simulink model "JABS"  (R2018b)
settings: Solver=FixedStepDiscrete  StartTime=0.0  StopTime=10.0  FixedStep=0.01  RelTol=1e-3
(part 2 of 2)

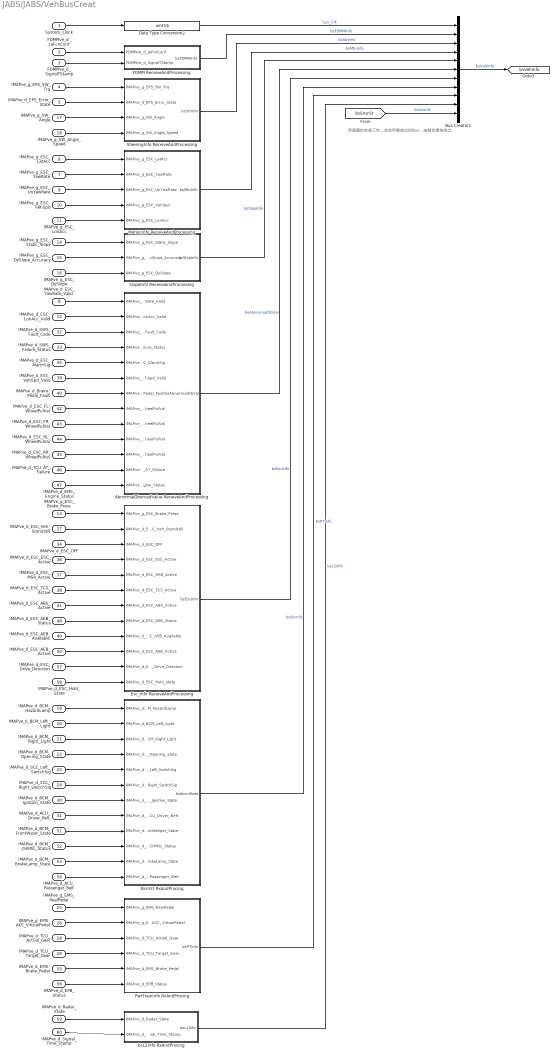
== system JABS/JABS/VehBusCreat ==
  note: 传感器的本身工作状态所集成出的Bus，由融合模块给出
  System_Clock : Inport
  FDMMve_d_JaFcnConf : Inport  Port=2
  FDMMve_d_SignalTStamp : Inport  Port=3
  IMAPve_g_EPS_SW_Trq : Inport  Port=4
  IMAPve_d_EPS_Error_State : Inport  Port=5
  IMAPve_g_ESC_LatAcc : Inport  Port=6
  IMAPve_g_ESC_YawRate : Inport  Port=7
  IMAPve_d_ESC_YawRate_Valid : Inport  Port=8
  IMAPve_g_ESC_UnYawRate : Inport  Port=9
  IMAPve_g_ESC_VehSpd : Inport  Port=10
  IMAPve_g_ESC_LonAcc : Inport  Port=11
  IMAPve_d_ESC_LonAcc_Valid : Inport  Port=12
  IMAPve_g_ESC_Brake_Press : Inport  Port=13
  IMAPve_g_ESC_Static_Slope : Inport  Port=14
  IMAPve_g_ESC_DySlope_Accuracy : Inport  Port=15
  IMAPve_g_ESC_DySlope : Inport  Port=16
  IMAPve_g_SW_Angle : Inport  Port=17
  IMAPve_g_SW_Angle_Speed : Inport  Port=18
  IMAPve_d_BCM_HazardLamp : Inport  Port=19
  IMAPve_d_BCM_Left_Light : Inport  Port=20
  IMAPve_d_BCM_Right_Light : Inport  Port=21
  IMAPve_d_BCM_Opening_State : Inport  Port=22
  IMAPve_d_SCC_Left_SwitchSig : Inport  Port=23
  IMAPve_d_SCC_Right_SwitchSig : Inport  Port=24
  IMAPve_g_EMS_RealPedal : Inport  Port=25
  IMAPve_g_EMS_ACC_VirtualPedal : Inport  Port=26
  IMAPve_d_ESC_Veh_Standstill : Inport  Port=27
  IMAPve_d_TCU_Actual_Gear : Inport  Port=28
  IMAPve_d_TCU_Target_Gear : Inport  Port=29
  IMAPve_d_BCM_Ignition_State : Inport  Port=30
  IMAPve_d_ACU_Driver_Belt : Inport  Port=31
  IMAPve_d_SWS_Fault_Code : Inport  Port=32
  IMAPve_d_SWS_Failure_Status : Inport  Port=33
  IMAPve_d_ESC_OFF : Inport  Port=34
  IMAPve_d_ESC_AlarmSig : Inport  Port=35
  IMAPve_d_ESC_ESC_Active : Inport  Port=36
  IMAPve_d_ESC_MSR_Active : Inport  Port=37
  IMAPve_d_ESC_TCS_Active : Inport  Port=38
  IMAPve_d_ESC_VehSpd_Valid : Inport  Port=39
  IMAPve_d_Brake_Pedal_Fault : Inport  Port=40
  IMAPve_d_ESC_ABS_Active : Inport  Port=41
  IMAPve_d_ESC_FL_WheelPulVal : Inport  Port=42
  IMAPve_d_ESC_FR_WheelPulVal : Inport  Port=43
  IMAPve_d_ESC_RL_WheelPulVal : Inport  Port=44
  IMAPve_d_ESC_RR_WheelPulVal : Inport  Port=45
  IMAPve_d_TCU_AT_Failure : Inport  Port=46
  IMAPve_d_EMS_Engine_Status : Inport  Port=47
  IMAPve_d_ESC_AEB_Status : Inport  Port=48
  IMAPve_d_ESC_AEB_Available : Inport  Port=49
  IMAPve_d_ESC_AEB_Active : Inport  Port=50
  IMAPve_d_BCM_FrontWiper_State : Inport  Port=51
  IMAPve_d_BCM_CHMSL_Status : Inport  Port=52
  IMAPve_d_BCM_BrakeLamp_State : Inport  Port=53
  IMAPve_d_ACU_Passenger_Belt : Inport  Port=54
  IMAPve_d_EMS_Brake_Pedal : Inport  Port=55
  IMAPve_d_EPB_Status : Inport  Port=56
  IMAPve_d_ESC_Drive_Direction : Inport  Port=57
  IMAPve_d_ESC_Hold_State : Inport  Port=58
  IMAPve_d_Radar_State : Inport  Port=59
  IMAPve_d_Signal_Time_Stamp : Inport  Port=60
  AbnormalObervedValue ReceiveAndProcessing : Subsystem
  BcmSt RxAndProcing : Subsystem
  Bus Creator1 : BusCreator  Inputs=11
  Data Type Conversion2 : DataTypeConversion  OutDataTypeStr=uint16
  Esc_Info ReceiveAndProcessing : Subsystem
  FDMM ReceiveAndProcessing : Subsystem
  MotionInfo ReceiveAndProcessing : Subsystem
  PwrTrainInfo RxAndProcing : Subsystem
  SlopeInfo ReceiveAndProcessing : Subsystem
  SteeringInfo ReceiveAndProcessing : Subsystem
  bsL2Info RxAndProcing : Subsystem
  tag scope: bsVehInfo=global
  wires:
  System_Clock/1 -> Data Type Conversion2/1
  IMAPve_d_EMS_Engine_Status/1 -> AbnormalObervedValue ReceiveAndProcessing/13(IMAPve_d_EMS_Engine_Status)
  IMAPve_d_TCU_AT_Failure/1 -> AbnormalObervedValue ReceiveAndProcessing/12(IMAPve_d_TCU_AT_Failure)
  SteeringInfo ReceiveAndProcessing/1(bsStrInfo) -> Bus Creator1/3  "bsStrInfo"
  IMAPve_d_Brake_Pedal_Fault/1 -> AbnormalObervedValue ReceiveAndProcessing/7(IMAPve_d_Brake_Pedal_Fault)
  IMAPve_d_ESC_FL_WheelPulVal/1 -> AbnormalObervedValue ReceiveAndProcessing/8(IMAPve_d_ESC_FL_WheelPulVal)
  IMAPve_g_SW_Angle/1 -> SteeringInfo ReceiveAndProcessing/3(IMAPve_g_SW_Angle)
  Esc_Info ReceiveAndProcessing/1(bsEscInfo) -> Bus Creator1/7  "bsEscInfo"
  IMAPve_d_EPS_Error_State/1 -> SteeringInfo ReceiveAndProcessing/2(IMAPve_d_EPS_Error_State)
  IMAPve_d_ESC_VehSpd_Valid/1 -> AbnormalObervedValue ReceiveAndProcessing/6(IMAPve_d_ESC_VehSpd_Valid)
  IMAPve_d_ESC_RL_WheelPulVal/1 -> AbnormalObervedValue ReceiveAndProcessing/10(IMAPve_d_ESC_RL_WheelPulVal)
  IMAPve_d_ESC_AlarmSig/1 -> AbnormalObervedValue ReceiveAndProcessing/5(IMAPve_d_ESC_AlarmSig)
  IMAPve_d_ESC_FR_WheelPulVal/1 -> AbnormalObervedValue ReceiveAndProcessing/9(IMAPve_d_ESC_FR_WheelPulVal)
  IMAPve_d_SWS_Failure_Status/1 -> AbnormalObervedValue ReceiveAndProcessing/4(IMAPve_d_SWS_Failure_Status)
  PwrTrainInfo RxAndProcing/1(bsPTInfo) -> Bus Creator1/9  "bsPTInfo"
  MotionInfo ReceiveAndProcessing/1(bsMtnInfo) -> Bus Creator1/4  "bsMtnInfo"
  IMAPve_g_SW_Angle_Speed/1 -> SteeringInfo ReceiveAndProcessing/4(IMAPve_g_SW_Angle_Speed)
  IMAPve_d_ESC_RR_WheelPulVal/1 -> AbnormalObervedValue ReceiveAndProcessing/11(IMAPve_d_ESC_RR_WheelPulVal)
  IMAPve_g_EMS_RealPedal/1 -> PwrTrainInfo RxAndProcing/1(IMAPve_g_EMS_RealPedal)
  IMAPve_g_EMS_ACC_VirtualPedal/1 -> PwrTrainInfo RxAndProcing/2(IMAPve_g_EMS_ACC_VirtualPedal)
  IMAPve_d_TCU_Actual_Gear/1 -> PwrTrainInfo RxAndProcing/3(IMAPve_d_TCU_Actual_Gear)
  IMAPve_d_SWS_Fault_Code/1 -> AbnormalObervedValue ReceiveAndProcessing/3(IMAPve_d_SWS_Fault_Code)
  IMAPve_d_EMS_Brake_Pedal/1 -> PwrTrainInfo RxAndProcing/5(IMAPve_d_EMS_Brake_Pedal)
  IMAPve_d_EPB_Status/1 -> PwrTrainInfo RxAndProcing/6(IMAPve_d_EPB_Status)
  IMAPve_g_EPS_SW_Trq/1 -> SteeringInfo ReceiveAndProcessing/1(IMAPve_g_EPS_SW_Trq)
  SlopeInfo ReceiveAndProcessing/1(bsSlopInfo) -> Bus Creator1/5  "bsSlopInfo"
  FDMM ReceiveAndProcessing/1(bsFDMMInfo) -> Bus Creator1/2  "bsFDMMInfo"
  IMAPve_d_ESC_LonAcc_Valid/1 -> AbnormalObervedValue ReceiveAndProcessing/2(IMAPve_d_ESC_LonAcc_Valid)
  IMAPve_d_ESC_YawRate_Valid/1 -> AbnormalObervedValue ReceiveAndProcessing/1(IMAPve_d_ESC_YawRate_Valid)
  IMAPve_d_TCU_Target_Gear/1 -> PwrTrainInfo RxAndProcing/4(IMAPve_d_TCU_Target_Gear)
  AbnormalObervedValue ReceiveAndProcessing/1(bsAbnormalObVal) -> Bus Creator1/6  "bsAbnormalObVal"
  Data Type Conversion2/1 -> Bus Creator1/1  "Sys_Clk"
  FDMMve_d_JaFcnConf/1 -> FDMM ReceiveAndProcessing/1(FDMMve_d_JaFcnConf)
  FDMMve_d_SignalTStamp/1 -> FDMM ReceiveAndProcessing/2(FDMMve_d_SignalTStamp)
  IMAPve_g_ESC_LatAcc/1 -> MotionInfo ReceiveAndProcessing/1(IMAPve_g_ESC_LatAcc)
  IMAPve_g_ESC_YawRate/1 -> MotionInfo ReceiveAndProcessing/2(IMAPve_g_ESC_YawRate)
  IMAPve_g_ESC_UnYawRate/1 -> MotionInfo ReceiveAndProcessing/3(IMAPve_g_ESC_UnYawRate)
  IMAPve_g_ESC_VehSpd/1 -> MotionInfo ReceiveAndProcessing/4(IMAPve_g_ESC_VehSpd)
  IMAPve_g_ESC_LonAcc/1 -> MotionInfo ReceiveAndProcessing/5(IMAPve_g_ESC_LonAcc)
  IMAPve_d_ESC_TCS_Active/1 -> Esc_Info ReceiveAndProcessing/6(IMAPve_d_ESC_TCS_Active)
  IMAPve_d_ESC_MSR_Active/1 -> Esc_Info ReceiveAndProcessing/5(IMAPve_d_ESC_MSR_Active)
  IMAPve_d_ESC_ABS_Active/1 -> Esc_Info ReceiveAndProcessing/7(IMAPve_d_ESC_ABS_Active)
  IMAPve_d_ESC_ESC_Active/1 -> Esc_Info ReceiveAndProcessing/4(IMAPve_d_ESC_ESC_Active)
  IMAPve_d_ESC_AEB_Status/1 -> Esc_Info ReceiveAndProcessing/8(IMAPve_d_ESC_AEB_Status)
  IMAPve_d_ESC_OFF/1 -> Esc_Info ReceiveAndProcessing/3(IMAPve_d_ESC_OFF)
  IMAPve_d_ESC_AEB_Available/1 -> Esc_Info ReceiveAndProcessing/9(IMAPve_d_ESC_AEB_Available)
  IMAPve_d_ESC_Veh_Standstill/1 -> Esc_Info ReceiveAndProcessing/2(IMAPve_d_ESC_Veh_Standstill)
  IMAPve_d_ESC_AEB_Active/1 -> Esc_Info ReceiveAndProcessing/10(IMAPve_d_ESC_AEB_Active)
  IMAPve_g_ESC_Brake_Press/1 -> Esc_Info ReceiveAndProcessing/1(IMAPve_g_ESC_Brake_Press)
  IMAPve_d_ESC_Drive_Direction/1 -> Esc_Info ReceiveAndProcessing/11(IMAPve_d_ESC_Drive_Direction)
  IMAPve_d_ESC_Hold_State/1 -> Esc_Info ReceiveAndProcessing/12(IMAPve_d_ESC_Hold_State)
  IMAPve_g_ESC_DySlope/1 -> SlopeInfo ReceiveAndProcessing/3(IMAPve_g_ESC_DySlope)
  IMAPve_g_ESC_DySlope_Accuracy/1 -> SlopeInfo ReceiveAndProcessing/2(IMAPve_g_ESC_DySlope_Accuracy)
  IMAPve_g_ESC_Static_Slope/1 -> SlopeInfo ReceiveAndProcessing/1(IMAPve_g_ESC_Static_Slope)
  IMAPve_d_BCM_HazardLamp/1 -> BcmSt RxAndProcing/1(IMAPve_d_BCM_HazardLamp)
  IMAPve_d_BCM_Left_Light/1 -> BcmSt RxAndProcing/2(IMAPve_d_BCM_Left_Light)
  IMAPve_d_BCM_Right_Light/1 -> BcmSt RxAndProcing/3(IMAPve_d_BCM_Right_Light)
  IMAPve_d_BCM_CHMSL_Status/1 -> BcmSt RxAndProcing/10(IMAPve_d_BCM_CHMSL_Status)
  IMAPve_d_BCM_BrakeLamp_State/1 -> BcmSt RxAndProcing/11(IMAPve_d_BCM_BrakeLamp_State)
  IMAPve_d_BCM_Opening_State/1 -> BcmSt RxAndProcing/4(IMAPve_d_BCM_Opening_State)
  IMAPve_d_SCC_Left_SwitchSig/1 -> BcmSt RxAndProcing/5(IMAPve_d_SCC_Left_SwitchSig)
  IMAPve_d_SCC_Right_SwitchSig/1 -> BcmSt RxAndProcing/6(IMAPve_d_SCC_Right_SwitchSig)
  IMAPve_d_BCM_Ignition_State/1 -> BcmSt RxAndProcing/7(IMAPve_d_BCM_Ignition_State)
  IMAPve_d_ACU_Driver_Belt/1 -> BcmSt RxAndProcing/8(IMAPve_d_ACU_Driver_Belt)
  IMAPve_d_ACU_Passenger_Belt/1 -> BcmSt RxAndProcing/12(IMAPve_d_ACU_Passenger_Belt)
  IMAPve_d_BCM_FrontWiper_State/1 -> BcmSt RxAndProcing/9(IMAPve_d_BCM_FrontWiper_State)
  BcmSt RxAndProcing/1(bsBcmState) -> Bus Creator1/8  "bsBcmSt"
  Bus Creator1/1 -> [bsVehInfo]  "bsVehInfo"
  IMAPve_d_Radar_State/1 -> bsL2Info RxAndProcing/1(IMAPve_d_Radar_State)
  IMAPve_d_Signal_Time_Stamp/1 -> bsL2Info RxAndProcing/2(IMAPve_d_Signal_Time_Stamp)
  bsL2Info RxAndProcing/1(bsL2Info) -> Bus Creator1/10  "bsL2Info"
  [bsSnsrSt] -> Bus Creator1/11  "bsSnsrSt"

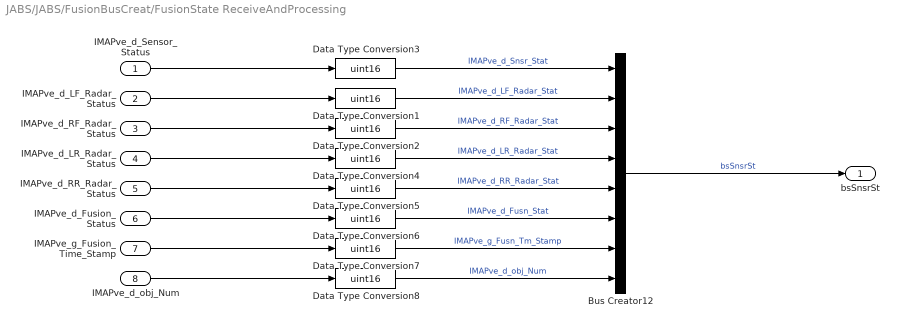
== system JABS/JABS/FusionBusCreat/FusionState ReceiveAndProcessing ==
  IMAPve_d_Sensor_Status : Inport
  IMAPve_d_LF_Radar_Status : Inport  Port=2
  IMAPve_d_RF_Radar_Status : Inport  Port=3
  IMAPve_d_LR_Radar_Status : Inport  Port=4
  IMAPve_d_RR_Radar_Status : Inport  Port=5
  IMAPve_d_Fusion_Status : Inport  Port=6
  IMAPve_g_Fusion_Time_Stamp : Inport  Port=7
  IMAPve_d_obj_Num : Inport  Port=8
  Bus Creator12 : BusCreator  Inputs=8
  Data Type Conversion{1..8} (8 alike) : DataTypeConversion  OutDataTypeStr=uint16
  bsSnsrSt : Outport
  wires:
  Data Type Conversion4/1 -> Bus Creator12/4  "IMAPve_d_LR_Radar_Stat"
  Data Type Conversion1/1 -> Bus Creator12/2  "IMAPve_d_LF_Radar_Stat"
  Data Type Conversion2/1 -> Bus Creator12/3  "IMAPve_d_RF_Radar_Stat"
  Data Type Conversion3/1 -> Bus Creator12/1  "IMAPve_d_Snsr_Stat"
  Data Type Conversion5/1 -> Bus Creator12/5  "IMAPve_d_RR_Radar_Stat"
  Data Type Conversion7/1 -> Bus Creator12/7  "IMAPve_g_Fusn_Tm_Stamp"
  Data Type Conversion6/1 -> Bus Creator12/6  "IMAPve_d_Fusn_Stat"
  Bus Creator12/1 -> bsSnsrSt/1  "bsSnsrSt"
  IMAPve_d_Sensor_Status/1 -> Data Type Conversion3/1
  IMAPve_d_LF_Radar_Status/1 -> Data Type Conversion1/1
  IMAPve_d_RF_Radar_Status/1 -> Data Type Conversion2/1
  IMAPve_d_LR_Radar_Status/1 -> Data Type Conversion4/1
  IMAPve_d_RR_Radar_Status/1 -> Data Type Conversion5/1
  IMAPve_d_Fusion_Status/1 -> Data Type Conversion6/1
  IMAPve_g_Fusion_Time_Stamp/1 -> Data Type Conversion7/1
  IMAPve_d_obj_Num/1 -> Data Type Conversion8/1
  Data Type Conversion8/1 -> Bus Creator12/8  "IMAPve_d_obj_Num"

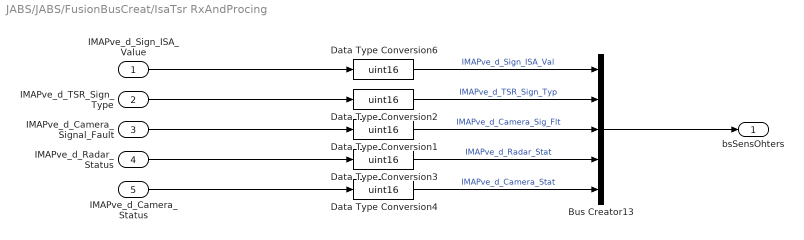
== system JABS/JABS/FusionBusCreat/IsaTsr RxAndProcing ==
  IMAPve_d_Sign_ISA_Value : Inport
  IMAPve_d_TSR_Sign_Type : Inport  Port=2
  IMAPve_d_Camera_Signal_Fault : Inport  Port=3
  IMAPve_d_Radar_Status : Inport  Port=4
  IMAPve_d_Camera_Status : Inport  Port=5
  Bus Creator13 : BusCreator  Inputs=5
  Data Type Conversion{1..4,6} (5 alike) : DataTypeConversion  OutDataTypeStr=uint16
  bsSensOhters : Outport
  wires:
  Data Type Conversion2/1 -> Bus Creator13/2  "IMAPve_d_TSR_Sign_Typ"
  Bus Creator13/1 -> bsSensOhters/1
  Data Type Conversion6/1 -> Bus Creator13/1  "IMAPve_d_Sign_ISA_Val"
  IMAPve_d_Sign_ISA_Value/1 -> Data Type Conversion6/1
  IMAPve_d_TSR_Sign_Type/1 -> Data Type Conversion2/1
  IMAPve_d_Camera_Signal_Fault/1 -> Data Type Conversion1/1
  Data Type Conversion1/1 -> Bus Creator13/3  "IMAPve_d_Camera_Sig_Flt"
  IMAPve_d_Radar_Status/1 -> Data Type Conversion3/1
  Data Type Conversion3/1 -> Bus Creator13/4  "IMAPve_d_Radar_Stat"
  IMAPve_d_Camera_Status/1 -> Data Type Conversion4/1
  Data Type Conversion4/1 -> Bus Creator13/5  "IMAPve_d_Camera_Stat"

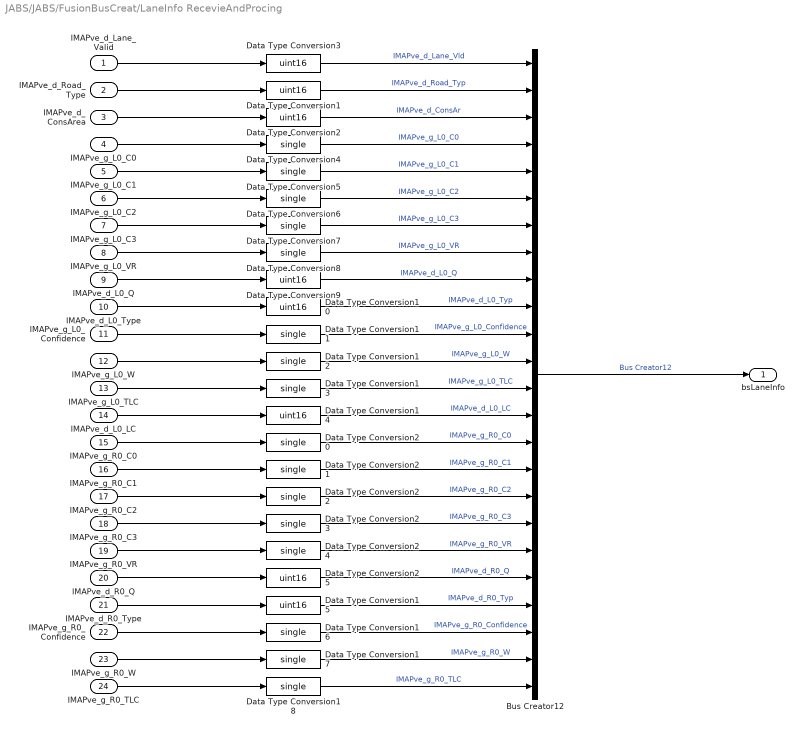
== system JABS/JABS/FusionBusCreat/LaneInfo RecevieAndProcing ==
  IMAPve_d_Lane_Valid : Inport
  IMAPve_d_Road_Type : Inport  Port=2
  IMAPve_d_ConsArea : Inport  Port=3
  IMAPve_g_L0_C0 : Inport  Port=4
  IMAPve_g_L0_C1 : Inport  Port=5
  IMAPve_g_L0_C2 : Inport  Port=6
  IMAPve_g_L0_C3 : Inport  Port=7
  IMAPve_g_L0_VR : Inport  Port=8
  IMAPve_d_L0_Q : Inport  Port=9
  IMAPve_d_L0_Type : Inport  Port=10
  IMAPve_g_L0_Confidence : Inport  Port=11
  IMAPve_g_L0_W : Inport  Port=12
  IMAPve_g_L0_TLC : Inport  Port=13
  IMAPve_d_L0_LC : Inport  Port=14
  IMAPve_g_R0_C0 : Inport  Port=15
  IMAPve_g_R0_C1 : Inport  Port=16
  IMAPve_g_R0_C2 : Inport  Port=17
  IMAPve_g_R0_C3 : Inport  Port=18
  IMAPve_g_R0_VR : Inport  Port=19
  IMAPve_d_R0_Q : Inport  Port=20
  IMAPve_d_R0_Type : Inport  Port=21
  IMAPve_g_R0_Confidence : Inport  Port=22
  IMAPve_g_R0_W : Inport  Port=23
  IMAPve_g_R0_TLC : Inport  Port=24
  Bus Creator12 : BusCreator  Inputs=24
  Data Type Conversion{1..3,9..10,14..15,25} (8 alike) : DataTypeConversion  OutDataTypeStr=uint16
  Data Type Conversion{4..8,11..13,16..18,20..24} (16 alike) : DataTypeConversion  OutDataTypeStr=single
  bsLaneInfo : Outport
  wires:
  Data Type Conversion20/1 -> Bus Creator12/15  "IMAPve_g_R0_C0"
  Data Type Conversion15/1 -> Bus Creator12/21  "IMAPve_d_R0_Typ"
  Data Type Conversion9/1 -> Bus Creator12/9  "IMAPve_d_L0_Q"
  Data Type Conversion18/1 -> Bus Creator12/24  "IMAPve_g_R0_TLC"
  Data Type Conversion14/1 -> Bus Creator12/14  "IMAPve_d_L0_LC"
  Data Type Conversion7/1 -> Bus Creator12/7  "IMAPve_g_L0_C3"
  Data Type Conversion6/1 -> Bus Creator12/6  "IMAPve_g_L0_C2"
  Data Type Conversion17/1 -> Bus Creator12/23  "IMAPve_g_R0_W"
  Data Type Conversion2/1 -> Bus Creator12/3  "IMAPve_d_ConsAr"
  Data Type Conversion21/1 -> Bus Creator12/16  "IMAPve_g_R0_C1"
  Data Type Conversion24/1 -> Bus Creator12/19  "IMAPve_g_R0_VR"
  Data Type Conversion10/1 -> Bus Creator12/10  "IMAPve_d_L0_Typ"
  Data Type Conversion23/1 -> Bus Creator12/18  "IMAPve_g_R0_C3"
  Data Type Conversion16/1 -> Bus Creator12/22  "IMAPve_g_R0_Confidence"
  Data Type Conversion22/1 -> Bus Creator12/17  "IMAPve_g_R0_C2"
  Data Type Conversion25/1 -> Bus Creator12/20  "IMAPve_d_R0_Q"
  Data Type Conversion1/1 -> Bus Creator12/2  "IMAPve_d_Road_Typ"
  Bus Creator12/1 -> bsLaneInfo/1  "Bus Creator12"
  Data Type Conversion12/1 -> Bus Creator12/12  "IMAPve_g_L0_W"
  Data Type Conversion3/1 -> Bus Creator12/1  "IMAPve_d_Lane_Vld"
  Data Type Conversion5/1 -> Bus Creator12/5  "IMAPve_g_L0_C1"
  Data Type Conversion8/1 -> Bus Creator12/8  "IMAPve_g_L0_VR"
  Data Type Conversion4/1 -> Bus Creator12/4  "IMAPve_g_L0_C0"
  Data Type Conversion13/1 -> Bus Creator12/13  "IMAPve_g_L0_TLC"
  Data Type Conversion11/1 -> Bus Creator12/11  "IMAPve_g_L0_Confidence"
  IMAPve_d_Lane_Valid/1 -> Data Type Conversion3/1
  IMAPve_d_Road_Type/1 -> Data Type Conversion1/1
  IMAPve_d_ConsArea/1 -> Data Type Conversion2/1
  IMAPve_g_L0_C0/1 -> Data Type Conversion4/1
  IMAPve_g_L0_C1/1 -> Data Type Conversion5/1
  IMAPve_g_L0_C2/1 -> Data Type Conversion6/1
  IMAPve_g_L0_C3/1 -> Data Type Conversion7/1
  IMAPve_g_L0_VR/1 -> Data Type Conversion8/1
  IMAPve_d_L0_Q/1 -> Data Type Conversion9/1
  IMAPve_d_L0_Type/1 -> Data Type Conversion10/1
  IMAPve_g_L0_Confidence/1 -> Data Type Conversion11/1
  IMAPve_g_L0_W/1 -> Data Type Conversion12/1
  IMAPve_g_L0_TLC/1 -> Data Type Conversion13/1
  IMAPve_d_L0_LC/1 -> Data Type Conversion14/1
  IMAPve_g_R0_C0/1 -> Data Type Conversion20/1
  IMAPve_g_R0_C1/1 -> Data Type Conversion21/1
  IMAPve_g_R0_C2/1 -> Data Type Conversion22/1
  IMAPve_g_R0_C3/1 -> Data Type Conversion23/1
  IMAPve_g_R0_VR/1 -> Data Type Conversion24/1
  IMAPve_d_R0_Q/1 -> Data Type Conversion25/1
  IMAPve_d_R0_Type/1 -> Data Type Conversion15/1
  IMAPve_g_R0_Confidence/1 -> Data Type Conversion16/1
  IMAPve_g_R0_W/1 -> Data Type Conversion17/1
  IMAPve_g_R0_TLC/1 -> Data Type Conversion18/1

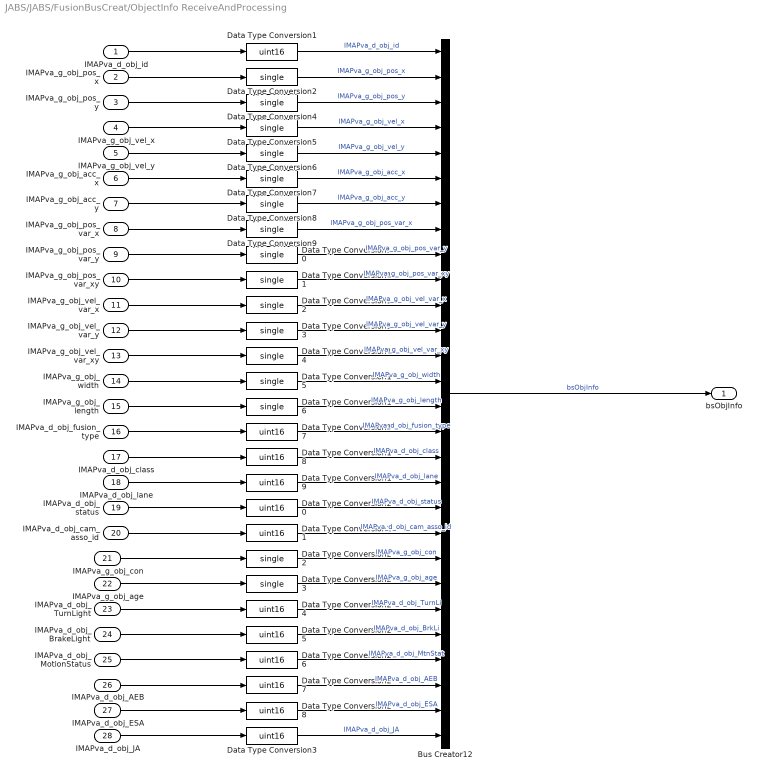
== system JABS/JABS/FusionBusCreat/ObjectInfo ReceiveAndProcessing ==
  IMAPva_d_obj_id : Inport
  IMAPva_g_obj_pos_x : Inport  Port=2
  IMAPva_g_obj_pos_y : Inport  Port=3
  IMAPva_g_obj_vel_x : Inport  Port=4
  IMAPva_g_obj_vel_y : Inport  Port=5
  IMAPva_g_obj_acc_x : Inport  Port=6
  IMAPva_g_obj_acc_y : Inport  Port=7
  IMAPva_g_obj_pos_var_x : Inport  Port=8
  IMAPva_g_obj_pos_var_y : Inport  Port=9
  IMAPva_g_obj_pos_var_xy : Inport  Port=10
  IMAPva_g_obj_vel_var_x : Inport  Port=11
  IMAPva_g_obj_vel_var_y : Inport  Port=12
  IMAPva_g_obj_vel_var_xy : Inport  Port=13
  IMAPva_g_obj_width : Inport  Port=14
  IMAPva_g_obj_length : Inport  Port=15
  IMAPva_d_obj_fusion_type : Inport  Port=16
  IMAPva_d_obj_class : Inport  Port=17
  IMAPva_d_obj_lane : Inport  Port=18
  IMAPva_d_obj_status : Inport  Port=19
  IMAPva_d_obj_cam_asso_id : Inport  Port=20
  IMAPva_g_obj_con : Inport  Port=21
  IMAPva_g_obj_age : Inport  Port=22
  IMAPva_d_obj_TurnLight : Inport  Port=23
  IMAPva_d_obj_BrakeLight : Inport  Port=24
  IMAPva_d_obj_MotionStatus : Inport  Port=25
  IMAPva_d_obj_AEB : Inport  Port=26
  IMAPva_d_obj_ESA : Inport  Port=27
  IMAPva_d_obj_JA : Inport  Port=28
  Bus Creator12 : BusCreator  Tag=RawSignalZip  Inputs=28
  Data Type Conversion{1,3,17..21,24..28} (12 alike) : DataTypeConversion  OutDataTypeStr=uint16
  Data Type Conversion{2,4..16,22..23} (16 alike) : DataTypeConversion  OutDataTypeStr=single
  bsObjInfo : Outport
  wires:
  Data Type Conversion14/1 -> Bus Creator12/13  "IMAPva_g_obj_vel_var_xy"
  Data Type Conversion6/1 -> Bus Creator12/5  "IMAPva_g_obj_vel_y"
  Data Type Conversion19/1 -> Bus Creator12/18  "IMAPva_d_obj_lane"
  Data Type Conversion10/1 -> Bus Creator12/9  "IMAPva_g_obj_pos_var_y"
  Data Type Conversion5/1 -> Bus Creator12/4  "IMAPva_g_obj_vel_x"
  Data Type Conversion25/1 -> Bus Creator12/24  "IMAPva_d_obj_BrkLi"
  Data Type Conversion27/1 -> Bus Creator12/26  "IMAPva_d_obj_AEB"
  Data Type Conversion26/1 -> Bus Creator12/25  "IMAPva_d_obj_MtnStat"
  Data Type Conversion4/1 -> Bus Creator12/3  "IMAPva_g_obj_pos_y"
  Data Type Conversion15/1 -> Bus Creator12/14  "IMAPva_g_obj_width"
  Data Type Conversion28/1 -> Bus Creator12/27  "IMAPva_d_obj_ESA"
  Data Type Conversion11/1 -> Bus Creator12/10  "IMAPva_g_obj_pos_var_xy"
  Data Type Conversion23/1 -> Bus Creator12/22  "IMAPva_g_obj_age"
  Data Type Conversion18/1 -> Bus Creator12/17  "IMAPva_d_obj_class"
  Data Type Conversion9/1 -> Bus Creator12/8  "IMAPva_g_obj_pos_var_x"
  Bus Creator12/1 -> bsObjInfo/1  "bsObjInfo"
  Data Type Conversion2/1 -> Bus Creator12/2  "IMAPva_g_obj_pos_x"
  Data Type Conversion21/1 -> Bus Creator12/20  "IMAPva_d_obj_cam_asso_id"
  Data Type Conversion7/1 -> Bus Creator12/6  "IMAPva_g_obj_acc_x"
  Data Type Conversion20/1 -> Bus Creator12/19  "IMAPva_d_obj_status"
  Data Type Conversion17/1 -> Bus Creator12/16  "IMAPva_d_obj_fusion_type"
  Data Type Conversion24/1 -> Bus Creator12/23  "IMAPva_d_obj_TurnLi"
  Data Type Conversion16/1 -> Bus Creator12/15  "IMAPva_g_obj_length"
  Data Type Conversion22/1 -> Bus Creator12/21  "IMAPva_g_obj_con"
  Data Type Conversion1/1 -> Bus Creator12/1  "IMAPva_d_obj_id"
  Data Type Conversion8/1 -> Bus Creator12/7  "IMAPva_g_obj_acc_y"
  Data Type Conversion13/1 -> Bus Creator12/12  "IMAPva_g_obj_vel_var_y"
  Data Type Conversion12/1 -> Bus Creator12/11  "IMAPva_g_obj_vel_var_x"
  IMAPva_d_obj_id/1 -> Data Type Conversion1/1
  IMAPva_g_obj_pos_x/1 -> Data Type Conversion2/1
  IMAPva_g_obj_pos_y/1 -> Data Type Conversion4/1
  IMAPva_g_obj_vel_x/1 -> Data Type Conversion5/1
  IMAPva_g_obj_vel_y/1 -> Data Type Conversion6/1
  IMAPva_g_obj_acc_x/1 -> Data Type Conversion7/1
  IMAPva_g_obj_acc_y/1 -> Data Type Conversion8/1
  IMAPva_g_obj_pos_var_x/1 -> Data Type Conversion9/1
  IMAPva_g_obj_pos_var_y/1 -> Data Type Conversion10/1
  IMAPva_g_obj_pos_var_xy/1 -> Data Type Conversion11/1
  IMAPva_g_obj_vel_var_x/1 -> Data Type Conversion12/1
  IMAPva_g_obj_vel_var_y/1 -> Data Type Conversion13/1
  IMAPva_g_obj_vel_var_xy/1 -> Data Type Conversion14/1
  IMAPva_g_obj_width/1 -> Data Type Conversion15/1
  IMAPva_g_obj_length/1 -> Data Type Conversion16/1
  IMAPva_d_obj_fusion_type/1 -> Data Type Conversion17/1
  IMAPva_d_obj_class/1 -> Data Type Conversion18/1
  IMAPva_d_obj_lane/1 -> Data Type Conversion19/1
  IMAPva_d_obj_status/1 -> Data Type Conversion20/1
  IMAPva_d_obj_cam_asso_id/1 -> Data Type Conversion21/1
  IMAPva_g_obj_con/1 -> Data Type Conversion22/1
  IMAPva_g_obj_age/1 -> Data Type Conversion23/1
  IMAPva_d_obj_TurnLight/1 -> Data Type Conversion24/1
  IMAPva_d_obj_BrakeLight/1 -> Data Type Conversion25/1
  IMAPva_d_obj_MotionStatus/1 -> Data Type Conversion26/1
  IMAPva_d_obj_AEB/1 -> Data Type Conversion27/1
  IMAPva_d_obj_ESA/1 -> Data Type Conversion28/1
  IMAPva_d_obj_JA/1 -> Data Type Conversion3/1
  Data Type Conversion3/1 -> Bus Creator12/28  "IMAPva_d_obj_JA"

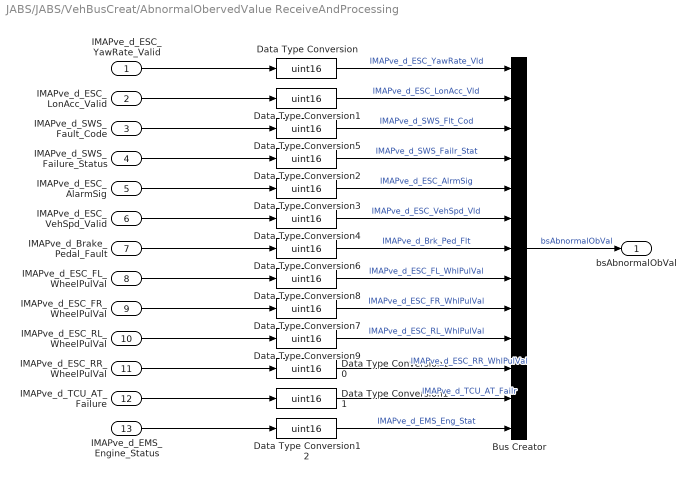
== system JABS/JABS/VehBusCreat/AbnormalObervedValue ReceiveAndProcessing ==
  IMAPve_d_ESC_YawRate_Valid : Inport
  IMAPve_d_ESC_LonAcc_Valid : Inport  Port=2
  IMAPve_d_SWS_Fault_Code : Inport  Port=3
  IMAPve_d_SWS_Failure_Status : Inport  Port=4
  IMAPve_d_ESC_AlarmSig : Inport  Port=5
  IMAPve_d_ESC_VehSpd_Valid : Inport  Port=6
  IMAPve_d_Brake_Pedal_Fault : Inport  Port=7
  IMAPve_d_ESC_FL_WheelPulVal : Inport  Port=8
  IMAPve_d_ESC_FR_WheelPulVal : Inport  Port=9
  IMAPve_d_ESC_RL_WheelPulVal : Inport  Port=10
  IMAPve_d_ESC_RR_WheelPulVal : Inport  Port=11
  IMAPve_d_TCU_AT_Failure : Inport  Port=12
  IMAPve_d_EMS_Engine_Status : Inport  Port=13
  Bus Creator : BusCreator  Inputs=13
  Data Type Conversion{,1..12} (13 alike) : DataTypeConversion  OutDataTypeStr=uint16
  bsAbnormalObVal : Outport
  wires:
  Data Type Conversion4/1 -> Bus Creator/6  "IMAPve_d_ESC_VehSpd_Vld"
  IMAPve_d_ESC_AlarmSig/1 -> Data Type Conversion3/1
  IMAPve_d_ESC_YawRate_Valid/1 -> Data Type Conversion/1
  IMAPve_d_ESC_LonAcc_Valid/1 -> Data Type Conversion1/1
  IMAPve_d_ESC_VehSpd_Valid/1 -> Data Type Conversion4/1
  Data Type Conversion8/1 -> Bus Creator/8  "IMAPve_d_ESC_FL_WhlPulVal"
  IMAPve_d_SWS_Fault_Code/1 -> Data Type Conversion5/1
  IMAPve_d_TCU_AT_Failure/1 -> Data Type Conversion11/1
  IMAPve_d_ESC_RR_WheelPulVal/1 -> Data Type Conversion10/1
  Data Type Conversion6/1 -> Bus Creator/7  "IMAPve_d_Brk_Ped_Flt"
  Data Type Conversion3/1 -> Bus Creator/5  "IMAPve_d_ESC_AlrmSig"
  Data Type Conversion/1 -> Bus Creator/1  "IMAPve_d_ESC_YawRate_Vld"
  Bus Creator/1 -> bsAbnormalObVal/1  "bsAbnormalObVal"
  Data Type Conversion7/1 -> Bus Creator/9  "IMAPve_d_ESC_FR_WhlPulVal"
  Data Type Conversion1/1 -> Bus Creator/2  "IMAPve_d_ESC_LonAcc_Vld"
  Data Type Conversion12/1 -> Bus Creator/13  "IMAPve_d_EMS_Eng_Stat"
  IMAPve_d_ESC_FL_WheelPulVal/1 -> Data Type Conversion8/1
  Data Type Conversion2/1 -> Bus Creator/4  "IMAPve_d_SWS_Failr_Stat"
  Data Type Conversion10/1 -> Bus Creator/11  "IMAPve_d_ESC_RR_WhlPulVal"
  Data Type Conversion11/1 -> Bus Creator/12  "IMAPve_d_TCU_AT_Failr"
  Data Type Conversion9/1 -> Bus Creator/10  "IMAPve_d_ESC_RL_WhlPulVal"
  IMAPve_d_ESC_FR_WheelPulVal/1 -> Data Type Conversion7/1
  Data Type Conversion5/1 -> Bus Creator/3  "IMAPve_d_SWS_Flt_Cod"
  IMAPve_d_SWS_Failure_Status/1 -> Data Type Conversion2/1
  IMAPve_d_Brake_Pedal_Fault/1 -> Data Type Conversion6/1
  IMAPve_d_ESC_RL_WheelPulVal/1 -> Data Type Conversion9/1
  IMAPve_d_EMS_Engine_Status/1 -> Data Type Conversion12/1

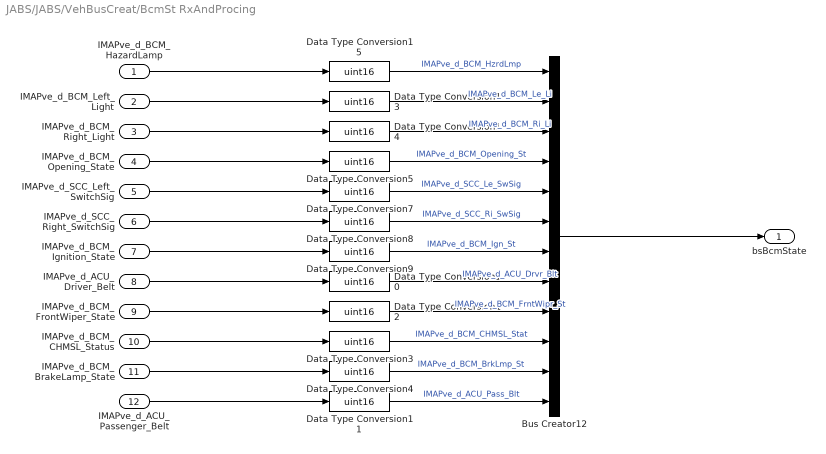
== system JABS/JABS/VehBusCreat/BcmSt RxAndProcing ==
  IMAPve_d_BCM_HazardLamp : Inport
  IMAPve_d_BCM_Left_Light : Inport  Port=2
  IMAPve_d_BCM_Right_Light : Inport  Port=3
  IMAPve_d_BCM_Opening_State : Inport  Port=4
  IMAPve_d_SCC_Left_SwitchSig : Inport  Port=5
  IMAPve_d_SCC_Right_SwitchSig : Inport  Port=6
  IMAPve_d_BCM_Ignition_State : Inport  Port=7
  IMAPve_d_ACU_Driver_Belt : Inport  Port=8
  IMAPve_d_BCM_FrontWiper_State : Inport  Port=9
  IMAPve_d_BCM_CHMSL_Status : Inport  Port=10
  IMAPve_d_BCM_BrakeLamp_State : Inport  Port=11
  IMAPve_d_ACU_Passenger_Belt : Inport  Port=12
  Bus Creator12 : BusCreator  Inputs=12
  Data Type Conversion{3..5,7..15} (12 alike) : DataTypeConversion  OutDataTypeStr=uint16
  bsBcmState : Outport
  wires:
  IMAPve_d_BCM_Left_Light/1 -> Data Type Conversion13/1
  Data Type Conversion10/1 -> Bus Creator12/8  "IMAPve_d_ACU_Drvr_Blt"
  Data Type Conversion14/1 -> Bus Creator12/3  "IMAPve_d_BCM_Ri_Li"
  Data Type Conversion3/1 -> Bus Creator12/10  "IMAPve_d_BCM_CHMSL_Stat"
  Data Type Conversion4/1 -> Bus Creator12/11  "IMAPve_d_BCM_BrkLmp_St"
  Data Type Conversion5/1 -> Bus Creator12/4  "IMAPve_d_BCM_Opening_St"
  Data Type Conversion12/1 -> Bus Creator12/9  "IMAPve_d_BCM_FrntWipr_St"
  IMAPve_d_BCM_BrakeLamp_State/1 -> Data Type Conversion4/1
  Data Type Conversion13/1 -> Bus Creator12/2  "IMAPve_d_BCM_Le_Li"
  IMAPve_d_BCM_CHMSL_Status/1 -> Data Type Conversion3/1
  Data Type Conversion9/1 -> Bus Creator12/7  "IMAPve_d_BCM_Ign_St"
  Data Type Conversion7/1 -> Bus Creator12/5  "IMAPve_d_SCC_Le_SwSig"
  Data Type Conversion15/1 -> Bus Creator12/1  "IMAPve_d_BCM_HzrdLmp"
  IMAPve_d_BCM_Opening_State/1 -> Data Type Conversion5/1
  IMAPve_d_SCC_Left_SwitchSig/1 -> Data Type Conversion7/1
  IMAPve_d_SCC_Right_SwitchSig/1 -> Data Type Conversion8/1
  Data Type Conversion11/1 -> Bus Creator12/12  "IMAPve_d_ACU_Pass_Blt"
  Data Type Conversion8/1 -> Bus Creator12/6  "IMAPve_d_SCC_Ri_SwSig"
  IMAPve_d_BCM_HazardLamp/1 -> Data Type Conversion15/1
  IMAPve_d_BCM_Right_Light/1 -> Data Type Conversion14/1
  IMAPve_d_BCM_Ignition_State/1 -> Data Type Conversion9/1
  IMAPve_d_ACU_Driver_Belt/1 -> Data Type Conversion10/1
  IMAPve_d_ACU_Passenger_Belt/1 -> Data Type Conversion11/1
  IMAPve_d_BCM_FrontWiper_State/1 -> Data Type Conversion12/1
  Bus Creator12/1 -> bsBcmState/1

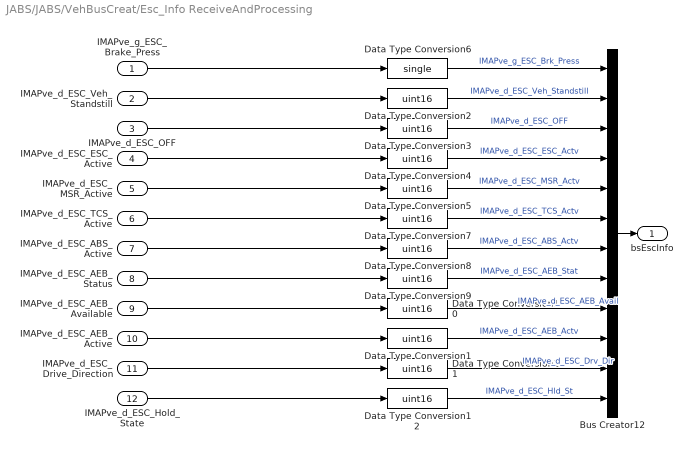
== system JABS/JABS/VehBusCreat/Esc_Info ReceiveAndProcessing ==
  IMAPve_g_ESC_Brake_Press : Inport
  IMAPve_d_ESC_Veh_Standstill : Inport  Port=2
  IMAPve_d_ESC_OFF : Inport  Port=3
  IMAPve_d_ESC_ESC_Active : Inport  Port=4
  IMAPve_d_ESC_MSR_Active : Inport  Port=5
  IMAPve_d_ESC_TCS_Active : Inport  Port=6
  IMAPve_d_ESC_ABS_Active : Inport  Port=7
  IMAPve_d_ESC_AEB_Status : Inport  Port=8
  IMAPve_d_ESC_AEB_Available : Inport  Port=9
  IMAPve_d_ESC_AEB_Active : Inport  Port=10
  IMAPve_d_ESC_Drive_Direction : Inport  Port=11
  IMAPve_d_ESC_Hold_State : Inport  Port=12
  Bus Creator12 : BusCreator  Inputs=12
  Data Type Conversion{1..5,7..12} (11 alike) : DataTypeConversion  OutDataTypeStr=uint16
  Data Type Conversion6 : DataTypeConversion  OutDataTypeStr=single
  bsEscInfo : Outport
  wires:
  Bus Creator12/1 -> bsEscInfo/1
  Data Type Conversion6/1 -> Bus Creator12/1  "IMAPve_g_ESC_Brk_Press"
  Data Type Conversion2/1 -> Bus Creator12/2  "IMAPve_d_ESC_Veh_Standstill"
  Data Type Conversion3/1 -> Bus Creator12/3  "IMAPve_d_ESC_OFF"
  Data Type Conversion4/1 -> Bus Creator12/4  "IMAPve_d_ESC_ESC_Actv"
  Data Type Conversion5/1 -> Bus Creator12/5  "IMAPve_d_ESC_MSR_Actv"
  Data Type Conversion7/1 -> Bus Creator12/6  "IMAPve_d_ESC_TCS_Actv"
  Data Type Conversion8/1 -> Bus Creator12/7  "IMAPve_d_ESC_ABS_Actv"
  Data Type Conversion9/1 -> Bus Creator12/8  "IMAPve_d_ESC_AEB_Stat"
  Data Type Conversion10/1 -> Bus Creator12/9  "IMAPve_d_ESC_AEB_Avail"
  Data Type Conversion1/1 -> Bus Creator12/10  "IMAPve_d_ESC_AEB_Actv"
  Data Type Conversion11/1 -> Bus Creator12/11  "IMAPve_d_ESC_Drv_Dir"
  Data Type Conversion12/1 -> Bus Creator12/12  "IMAPve_d_ESC_Hld_St"
  IMAPve_g_ESC_Brake_Press/1 -> Data Type Conversion6/1
  IMAPve_d_ESC_Veh_Standstill/1 -> Data Type Conversion2/1
  IMAPve_d_ESC_OFF/1 -> Data Type Conversion3/1
  IMAPve_d_ESC_ESC_Active/1 -> Data Type Conversion4/1
  IMAPve_d_ESC_MSR_Active/1 -> Data Type Conversion5/1
  IMAPve_d_ESC_TCS_Active/1 -> Data Type Conversion7/1
  IMAPve_d_ESC_ABS_Active/1 -> Data Type Conversion8/1
  IMAPve_d_ESC_AEB_Status/1 -> Data Type Conversion9/1
  IMAPve_d_ESC_AEB_Available/1 -> Data Type Conversion10/1
  IMAPve_d_ESC_AEB_Active/1 -> Data Type Conversion1/1
  IMAPve_d_ESC_Drive_Direction/1 -> Data Type Conversion11/1
  IMAPve_d_ESC_Hold_State/1 -> Data Type Conversion12/1

== system JABS/JABS/VehBusCreat/FDMM ReceiveAndProcessing ==
  FDMMve_d_JaFcnConf : Inport
  FDMMve_d_SignalTStamp : Inport  Port=2
  Bus Creator12 : BusCreator  Inputs=2
  Data Type Conversion2 : DataTypeConversion  OutDataTypeStr=uint16
  Data Type Conversion6 : DataTypeConversion  OutDataTypeStr=uint16
  bsFDMMInfo : Outport
  wires:
  Bus Creator12/1 -> bsFDMMInfo/1
  Data Type Conversion2/1 -> Bus Creator12/2  "FDMMve_d_SigTStamp"
  Data Type Conversion6/1 -> Bus Creator12/1  "FDMMve_d_JaFcnConf"
  FDMMve_d_JaFcnConf/1 -> Data Type Conversion6/1
  FDMMve_d_SignalTStamp/1 -> Data Type Conversion2/1

== system JABS/JABS/VehBusCreat/MotionInfo ReceiveAndProcessing ==
  IMAPve_g_ESC_LatAcc : Inport
  IMAPve_g_ESC_YawRate : Inport  Port=2
  IMAPve_g_ESC_UnYawRate : Inport  Port=3
  IMAPve_g_ESC_VehSpd : Inport  Port=4
  IMAPve_g_ESC_LonAcc : Inport  Port=5
  Bus Creator12 : BusCreator  Inputs=5
  Data Type Conversion{1..5} (5 alike) : DataTypeConversion  OutDataTypeStr=single
  bsMtnInfo : Outport
  wires:
  Data Type Conversion4/1 -> Bus Creator12/4  "IMAPve_g_ESC_VehSpd"
  Data Type Conversion3/1 -> Bus Creator12/1  "IMAPve_g_ESC_LatAcc"
  Data Type Conversion1/1 -> Bus Creator12/2  "IMAPve_g_ESC_YawRate"
  Data Type Conversion2/1 -> Bus Creator12/3  "IMAPve_g_ESC_UnYawRate"
  Data Type Conversion5/1 -> Bus Creator12/5  "IMAPve_g_ESC_LonAcc"
  IMAPve_g_ESC_LatAcc/1 -> Data Type Conversion3/1
  IMAPve_g_ESC_YawRate/1 -> Data Type Conversion1/1
  IMAPve_g_ESC_UnYawRate/1 -> Data Type Conversion2/1
  IMAPve_g_ESC_VehSpd/1 -> Data Type Conversion4/1
  IMAPve_g_ESC_LonAcc/1 -> Data Type Conversion5/1
  Bus Creator12/1 -> bsMtnInfo/1

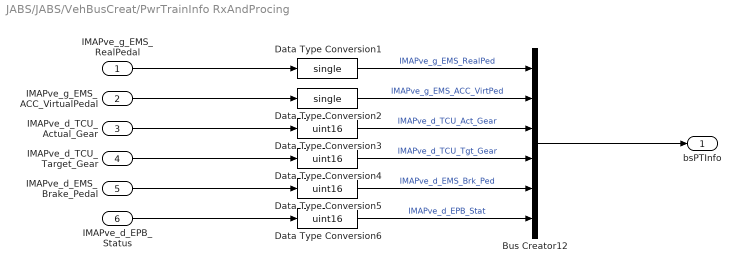
== system JABS/JABS/VehBusCreat/PwrTrainInfo RxAndProcing ==
  IMAPve_g_EMS_RealPedal : Inport
  IMAPve_g_EMS_ACC_VirtualPedal : Inport  Port=2
  IMAPve_d_TCU_Actual_Gear : Inport  Port=3
  IMAPve_d_TCU_Target_Gear : Inport  Port=4
  IMAPve_d_EMS_Brake_Pedal : Inport  Port=5
  IMAPve_d_EPB_Status : Inport  Port=6
  Bus Creator12 : BusCreator  Inputs=6
  Data Type Conversion1 : DataTypeConversion  OutDataTypeStr=single
  Data Type Conversion2 : DataTypeConversion  OutDataTypeStr=single
  Data Type Conversion{3..6} (4 alike) : DataTypeConversion  OutDataTypeStr=uint16
  bsPTInfo : Outport
  wires:
  Data Type Conversion6/1 -> Bus Creator12/6  "IMAPve_d_EPB_Stat"
  Data Type Conversion1/1 -> Bus Creator12/1  "IMAPve_g_EMS_RealPed"
  IMAPve_g_EMS_RealPedal/1 -> Data Type Conversion1/1
  Data Type Conversion5/1 -> Bus Creator12/5  "IMAPve_d_EMS_Brk_Ped"
  Data Type Conversion4/1 -> Bus Creator12/4  "IMAPve_d_TCU_Tgt_Gear"
  Data Type Conversion2/1 -> Bus Creator12/2  "IMAPve_g_EMS_ACC_VirtPed"
  Data Type Conversion3/1 -> Bus Creator12/3  "IMAPve_d_TCU_Act_Gear"
  Bus Creator12/1 -> bsPTInfo/1
  IMAPve_g_EMS_ACC_VirtualPedal/1 -> Data Type Conversion2/1
  IMAPve_d_TCU_Actual_Gear/1 -> Data Type Conversion3/1
  IMAPve_d_TCU_Target_Gear/1 -> Data Type Conversion4/1
  IMAPve_d_EMS_Brake_Pedal/1 -> Data Type Conversion5/1
  IMAPve_d_EPB_Status/1 -> Data Type Conversion6/1

== system JABS/JABS/VehBusCreat/SlopeInfo ReceiveAndProcessing ==
  IMAPve_g_ESC_Static_Slope : Inport
  IMAPve_g_ESC_DySlope_Accuracy : Inport  Port=2
  IMAPve_g_ESC_DySlope : Inport  Port=3
  Bus Creator12 : BusCreator  Inputs=3
  Data Type Conversion1 : DataTypeConversion  OutDataTypeStr=single
  Data Type Conversion2 : DataTypeConversion  OutDataTypeStr=single
  Data Type Conversion6 : DataTypeConversion  OutDataTypeStr=single
  bsSlopInfo : Outport
      settings: AttributesFormatString=Disable Action: %<OutputWhenDisabled>
  wires:
  Bus Creator12/1 -> bsSlopInfo/1  "Bus Creator12"
  Data Type Conversion1/1 -> Bus Creator12/2  "IMAPve_g_ESC_DySlop_Accuracy"
  Data Type Conversion6/1 -> Bus Creator12/1  "IMAPve_g_ESC_Stac_Slop"
  Data Type Conversion2/1 -> Bus Creator12/3  "IMAPve_g_ESC_DySlop"
  IMAPve_g_ESC_DySlope/1 -> Data Type Conversion2/1
  IMAPve_g_ESC_DySlope_Accuracy/1 -> Data Type Conversion1/1
  IMAPve_g_ESC_Static_Slope/1 -> Data Type Conversion6/1

== system JABS/JABS/VehBusCreat/SteeringInfo ReceiveAndProcessing ==
  IMAPve_g_EPS_SW_Trq : Inport
  IMAPve_d_EPS_Error_State : Inport  Port=2
  IMAPve_g_SW_Angle : Inport  Port=3
  IMAPve_g_SW_Angle_Speed : Inport  Port=4
  Bus Creator12 : BusCreator  Inputs=4
  Data Type Conversion1 : DataTypeConversion  OutDataTypeStr=uint16
  Data Type Conversion2 : DataTypeConversion  OutDataTypeStr=single
  Data Type Conversion3 : DataTypeConversion  OutDataTypeStr=single
  Data Type Conversion5 : DataTypeConversion  OutDataTypeStr=single
  bsStrInfo : Outport
  wires:
  Data Type Conversion5/1 -> Bus Creator12/1  "IMAPve_g_EPS_SW_Trq"
  Data Type Conversion3/1 -> Bus Creator12/4  "IMAPve_g_SW_Ang_Spd"
  Data Type Conversion2/1 -> Bus Creator12/3  "IMAPve_g_SW_Ang"
  Data Type Conversion1/1 -> Bus Creator12/2  "IMAPve_d_EPS_Err_St"
  Bus Creator12/1 -> bsStrInfo/1
  IMAPve_g_EPS_SW_Trq/1 -> Data Type Conversion5/1
  IMAPve_d_EPS_Error_State/1 -> Data Type Conversion1/1
  IMAPve_g_SW_Angle/1 -> Data Type Conversion2/1
  IMAPve_g_SW_Angle_Speed/1 -> Data Type Conversion3/1

== system JABS/JABS/VehBusCreat/bsL2Info RxAndProcing ==
  IMAPve_d_Radar_State : Inport
  IMAPve_d_Signal_Time_Stamp : Inport  Port=2
  Bus Creator : BusCreator  Inputs=2
  Data Type Conversion1 : DataTypeConversion  OutDataTypeStr=uint32
  Data Type Conversion6 : DataTypeConversion  OutDataTypeStr=uint16
  bsL2Info : Outport
  wires:
  IMAPve_d_Signal_Time_Stamp/1 -> Data Type Conversion1/1
  Data Type Conversion1/1 -> Bus Creator/2  "IMAPve_d_Sig_Tm_Stamp"
  Data Type Conversion6/1 -> Bus Creator/1  "IMAPve_d_Radar_St"
  Bus Creator/1 -> bsL2Info/1  "bsL2Info"
  IMAPve_d_Radar_State/1 -> Data Type Conversion6/1
